simulink model "Arrays1"  (Simulink 5.0)
settings: Solver=FixedStepDiscrete  StartTime=0.0  StopTime=10000.0  RelTol=1e-3
settings Model: Creator=scaife  LastModifiedBy=scaife  ExtModeAutoUpdateStatusClock=off

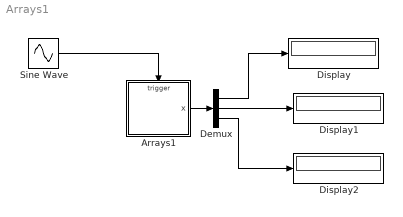
== system Arrays1 ==
  Arrays1 : Stateflow chart
  Demux : Demux  Outputs=3
  Display : Display
  Display1 : Display
  Display2 : Display
  Sine Wave : Sin  SampleTime=0
  wires:
  Sine Wave/1 -> Arrays1/Trigger
  Arrays1/1(x) -> Demux/1
  Demux/1 -> Display/1
  Demux/2 -> Display1/1
  Demux/3 -> Display2/1

== stateflow chart Arrays1 ==
  state A/
    en:x[1]++;
  state B/
    en:x[2]++;
  state C/
    en:x[3]++;
  (default) -> A
  A -> B : E
  B -> C : E
  C -> A : E
  data: x output int32 size=3 [0..100] =1
  events: E input RISING_EDGE_EVENT
